simulink model "TestingQuestFSW"  (R2025b)
settings: Solver=FixedStepAuto  StartTime=0.0  StopTime=10  FixedStep=0.1  RelTol=1e-3
libraries: sharedutil x1, sFunctionLibrary x1
settings Model: Creator=AdamY  LastModifiedBy=AdamY

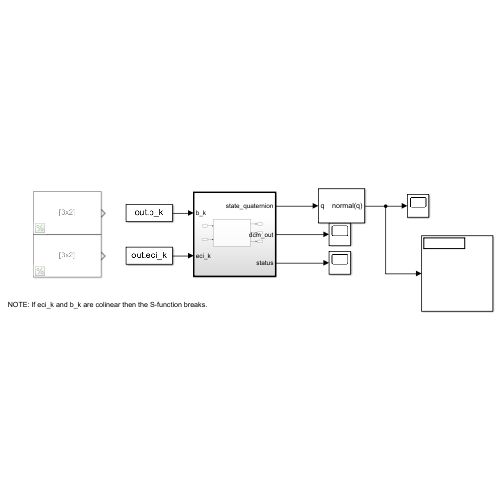
[thumbnail: Simulink's stored preview of the top-level diagram]
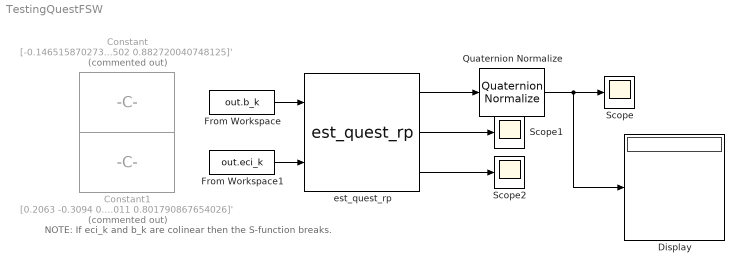
== system TestingQuestFSW ==
  note: NOTE: If eci_k and b_k are colinear then the S-function breaks.
  Constant : Constant  Commented=on  Value=[-0.146515870273397 -0.380940289663793 0.912917080281060; 0.346003335147385 0.317941852747502 0.882720040748125]'  OutDataTypeStr=single
  Constant1 : Constant  Commented=on  Value=[0.2063 -0.3094 0.9283; 0.267296955505015 0.534493912149011 0.801790867654026]'  OutDataTypeStr=single
  Display : Display
  From Workspace : FromWorkspace  VariableName=out.b_k
  From Workspace1 : FromWorkspace  VariableName=out.eci_k
  Quaternion Normalize : sharedutil/Quaternion Normalize  aMode=aMode
  Scope : Scope
      settings: ActiveDisplayYMinimum=-0.1526709012687206  ActiveDisplayYMaximum=1.0850297920405865
  Scope1 : Scope
      settings: ActiveDisplayYMinimum=-1  ActiveDisplayYMaximum=1
  Scope2 : Scope
      settings: ActiveDisplayYMinimum=-1  ActiveDisplayYMaximum=1  DataLoggingVariableName=ScopeData2
  est_quest_rp : sFunctionLibrary/est_quest_rp  SystemSampleTime=-1  VariantActivationTime=update diagram  EmptyChoice=off  PassThrough=off  PassThroughVariantControl=(default)  EmptyChoiceVariantControl=(default)  AllowFlexibleInterface=on  Latency=0  AutoFrameSizeCalculation=off
  wires:
  est_quest_rp/1 -> Quaternion Normalize/1
  est_quest_rp/2 -> Scope1/1
  est_quest_rp/3 -> Scope2/1
  Quaternion Normalize/1 -> Display/1, Scope/1
  From Workspace/1 -> est_quest_rp/1
  From Workspace1/1 -> est_quest_rp/2
